simulink model "untitled"  (R2024b)
settings: Solver=VariableStepAuto  StartTime=0.0  StopTime=10.0  RelTol=1e-3
settings Model: Creator=Sagar  LastModifiedBy=Sagar

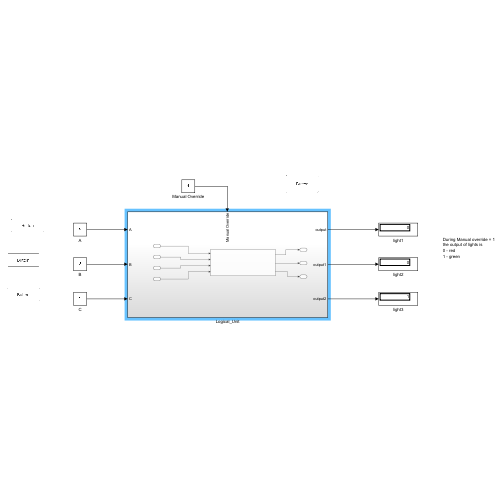
[thumbnail: Simulink's stored preview of the top-level diagram]
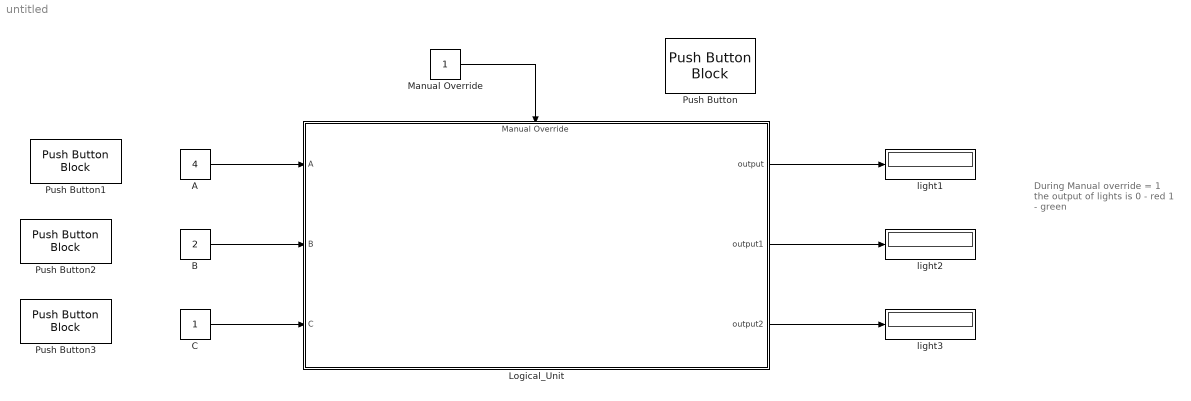
== system untitled ==
  note: During Manual override = 1
      | the output of lights is
      | 0 - red
      | 1 - green
  A : Constant  Value=4
  B : Constant  Value=2
  C : Constant
  Logical_Unit : Subsystem
      settings: PortSchema="{\"entries\":[{\"content\":{\"sides\":[{\"content\":{\"connectorIds\":[\"In1\",\"In2\",\"In3\"]},\"type\":\"ConnectorPlacement.EquallySpacedRectSide\",\"uuid\":\"8855ce6d-d1ff-4d7f-a3df-67bdf88ab5f5\"},{\"content\":{\"connectorIds\":[\"Out1\",\"Out2\",\"Out3\"],\"side\":\"RIGHT\"},\"type\":\"ConnectorPlacement.EquallySpacedRectSide\",\"uuid\":\"52f56ae2-25c7-4c8f-a76f-4a07a3778792\"},{\"content\":{\"connectorIds\":[\"In4\"],\"side\":\"TOP\"},\"type\":\"ConnectorPlacement.EquallySpacedRectSide\",\"uuid\":\"7fe2cf04-5da7-44c6-9157-4fd5825aeae5\"}]},\"type\":\"ConnectorPlacement.EquallySpacedConnector\",\"uuid\":\"d49c1084-20b5-4dd5-a2b8-171e20c1de77\"}],\"packageUris\":[\"http://schema.mathworks.com/mf0/Connector/R2020b\"],\"version\":\"1.0\"}"
  Manual Override : Constant
  Push Button : PushButtonBlock  OnValue=0  ButtonType=Latch  OffValue=1.000000
  Push Button1 : PushButtonBlock  OnValue=99  ButtonType=Latch  OffValue=4.000000
  Push Button2 : PushButtonBlock  OnValue=99  ButtonType=Latch
  Push Button3 : PushButtonBlock  ButtonType=Latch
  light1 : Display
  light2 : Display
  light3 : Display
  wires:
  Logical_Unit/1(output) -> light1/1
  A/1 -> Logical_Unit/1(A)
  B/1 -> Logical_Unit/2(B)
  C/1 -> Logical_Unit/3(C)
  Manual Override/1 -> Logical_Unit/4(Manual Override)
  Logical_Unit/2(output1) -> light2/1
  Logical_Unit/3(output2) -> light3/1

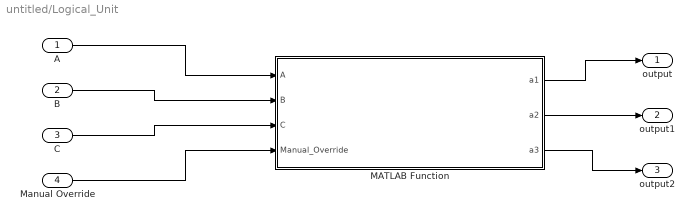
== system untitled/Logical_Unit ==
  A : Inport
  B : Inport  Port=2
  C : Inport  Port=3
  Manual Override : Inport  Port=4
  MATLAB Function : MATLAB Function  TreatAsAtomicUnit=on
  output : Outport
  output1 : Outport  Port=2
  output2 : Outport  Port=3
  wires:
  A/1 -> MATLAB Function/1(A)
  B/1 -> MATLAB Function/2(B)
  C/1 -> MATLAB Function/3(C)
  Manual Override/1 -> MATLAB Function/4(Manual_Override)
  MATLAB Function/1(a1) -> output/1
  MATLAB Function/2(a2) -> output1/1
  MATLAB Function/3(a3) -> output2/1

== matlab function untitled/Logical_Unit/MATLAB Function ==
  data: A input; a1 output; B input; C input; Manual_Override input; a2 output; a3 output
function [a1, a2, a3] = fcn(A, B, C, Manual_Override)
    % Initialize outputs
    a1 = 0;
    a2 = 0;
    a3 = 0;

    % Manual Override Mode
    if Manual_Override == 1
        if A == 99
            a1 = 1;
            a2 = 0;
            a3 = 0;
        elseif B == 99
            a1 = 0;
            a2 = 1;
            a3 = 0;
        elseif C == 99
            a1 = 0;
            a2 = 0;
            a3 = 1;
        end
    else
        % Automatic Mode (Traffic Light Logic)
        if A > B && B > C
            disp("A = green");
            disp("B = yellow");
            disp("C = red");
            a1 = 1; % Green
            a2 = 2; % Yellow
            a3 = 3; % Red
        elseif B > C && C > A
            disp("A = red");
            disp("B = green");
            disp("C = yellow");
            a1 = 3; % Red
            a2 = 1; % Green
            a3 = 2; % Yellow
        elseif C > A && A > B
            disp("A = yellow");
            disp("B = red");
            disp("C = green");
            a1 = 2; % Yellow
            a2 = 3; % Red
            a3 = 1; % Green
        else
            disp("Invalid input or equal values.");
        end
    end
end
